simulink model "z_Ralenti_BO_End"  (R2024b)
settings: Solver=VariableStepAuto  StartTime=0.0  StopTime=10.0  RelTol=1e-3
undefined symbols (not defined in the file): AaNeTest, AAopti, Copti, gam, J, Kv, Mim0, N0, NeTest, NeTimeTest, nv_remp, P0, Pamb, PcolNeTest, PRcrit, Rair, SectionBpNeTest, table_rdt_AA, Tamb, Vcyl, vect_delta_AA
settings Model: Creator=a030141  LastModifiedBy=ramse
settings DebuggingCC: UnderspecifiedInitializationDetection=Classic  MergeDetectMultiDrivingBlocksExec=none
settings ModelReferenceCC: PropagateSignalLabelsOutOfModel=off

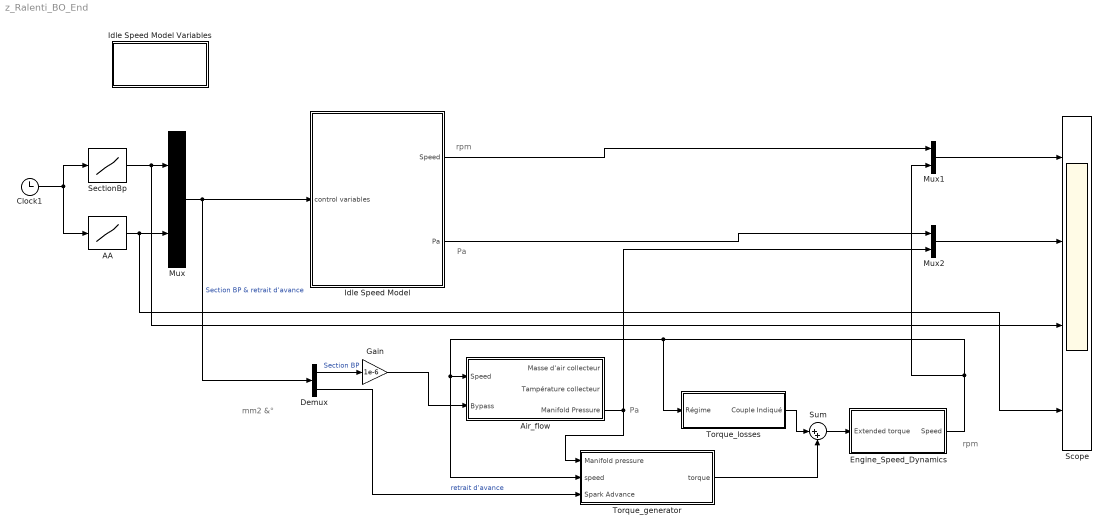
== system z_Ralenti_BO_End ==
  note: Pa
  note: rpm
  note: mm2 &°
  note: rpm
  note: Pa
  AA : Lookup  InputValues=NeTimeTest  Table=AaNeTest
  Air_flow : Subsystem
  Clock1 : Clock
  Demux : Demux  Outputs=2
  Engine_Speed_Dynamics : Subsystem
  Gain : Gain  Gain=1e-6
  Idle Speed Model : Subsystem
      mask Display: disp('ENGINE MODEL\nLF -> event stroke')
  Idle Speed Model Variables : Subsystem
      mask Display: disp('Load\nDisturbances')
  Mux : Mux  Inputs=2
      settings: DisplayOption=signals
  Mux1 : Mux  Inputs=2
  Mux2 : Mux  Inputs=2
  Scope : Scope  NumInputPorts=4
  SectionBp : Lookup  InputValues=NeTimeTest  Table=SectionBpNeTest
  Sum : Sum  Inputs=|++
  Torque_generator : Subsystem
  Torque_losses : Subsystem
  wires:
  Mux/1 -> Idle Speed Model/1(control variables), Demux/1  "Section BP & retrait d'avance"
  SectionBp/1 -> Mux/1, Scope/3
  AA/1 -> Mux/2, Scope/4
  Clock1/1 -> SectionBp/1, AA/1
  Idle Speed Model/1(Speed) -> Mux1/1
  Mux1/1 -> Scope/1
  Idle Speed Model/2(Pa) -> Mux2/1
  Mux2/1 -> Scope/2
  Demux/1 -> Gain/1  "Section BP"
  Demux/2 -> Torque_generator/3(Spark Advance)  "retrait d'avance"
  Air_flow/3(Manifold Pressure) -> Torque_generator/1(Manifold pressure), Mux2/2
  Engine_Speed_Dynamics/1(Speed) -> Mux1/2, Torque_losses/1(Régime), Torque_generator/2(speed), Air_flow/1(Speed)
  Gain/1 -> Air_flow/2(Bypass)
  Torque_losses/1(Couple Indiqué) -> Sum/1
  Torque_generator/1(torque) -> Sum/2
  Sum/1 -> Engine_Speed_Dynamics/1(Extended torque)

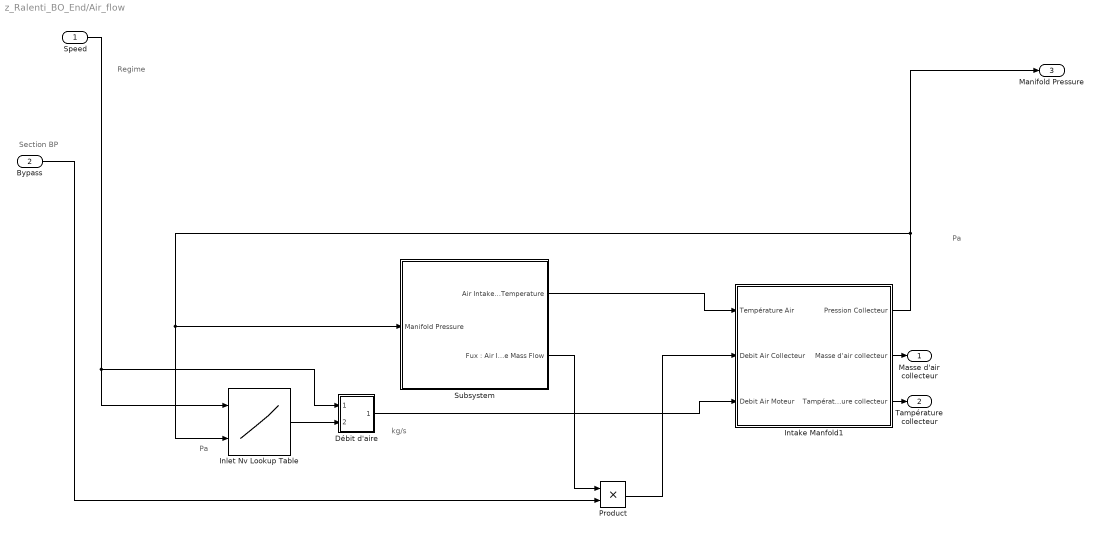
== system z_Ralenti_BO_End/Air_flow ==
  note: Section BP
  note: Regime
  note: Pa
  note: Pa
  note: kg/s
  Speed : Inport
  Bypass : Inport  Port=2
  Débit d'aire : Subsystem
  Inlet Nv Lookup Table : Lookup2D  RowIndex=Ne_remp  ColumnIndex=Pcol_remp  Table=nv_remp
  Intake Manfold1 : Subsystem
  Product : Product
  Subsystem : Subsystem
  Masse d'air collecteur : Outport
  Tampérature collecteur : Outport  Port=2
  Manifold Pressure : Outport  Port=3
  wires:
  Débit d'aire/1(Debit Air Moteur) -> Intake Manfold1/3(Debit Air Moteur)
  Speed/1 -> Débit d'aire/1(In1), Inlet Nv Lookup Table/1
  Intake Manfold1/2(Masse d'air collecteur) -> Masse d'air collecteur/1
  Subsystem/1(Air Intake Temperature) -> Intake Manfold1/1(Température Air)
  Subsystem/2("Fux : Air Intake Mass Flow") -> Product/1
  Inlet Nv Lookup Table/1 -> Débit d'aire/2(In2)
  Product/1 -> Intake Manfold1/2(Debit Air Collecteur)
  Intake Manfold1/1(Pression Collecteur) -> Manifold Pressure/1, Inlet Nv Lookup Table/2, Subsystem/1(Manifold Pressure)
  Bypass/1 -> Product/2
  Intake Manfold1/3(Tampérature collecteur) -> Tampérature collecteur/1

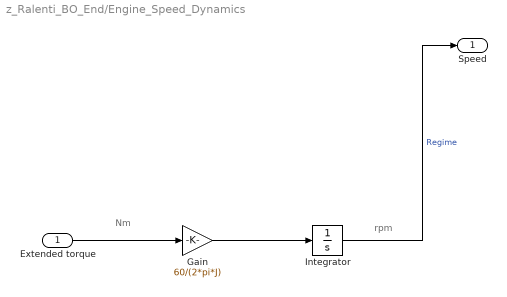
== system z_Ralenti_BO_End/Engine_Speed_Dynamics ==
  note: rpm
  note: Nm
  Extended torque : Inport
  Gain : Gain  Gain=60/(2*pi*J)
  Integrator : Integrator  InitialCondition=N0
  Speed : Outport
  wires:
  Gain/1 -> Integrator/1
  Extended torque/1 -> Gain/1
  Integrator/1 -> Speed/1  "Regime"

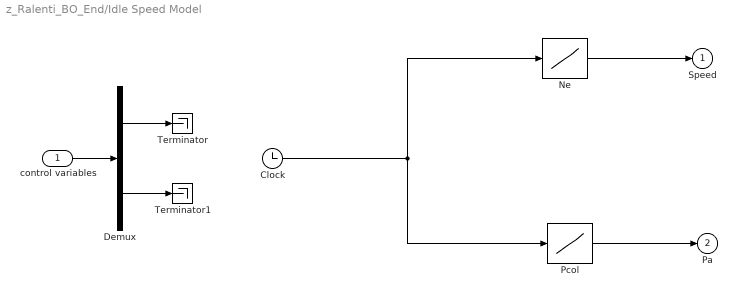
== system z_Ralenti_BO_End/Idle Speed Model ==
  control variables : Inport
  Clock : Clock
  Demux : Demux  Outputs=2
      settings: DisplayOption=none
  Ne : Lookup  InputValues=NeTimeTest  Table=NeTest
  Pcol : Lookup  InputValues=NeTimeTest  Table=PcolNeTest
  Terminator : Terminator
  Terminator1 : Terminator
  Speed : Outport
  Pa : Outport  Port=2
  wires:
  Demux/1 -> Terminator/1
  control variables/1 -> Demux/1
  Ne/1 -> Speed/1
  Pcol/1 -> Pa/1
  Clock/1 -> Ne/1, Pcol/1
  Demux/2 -> Terminator1/1

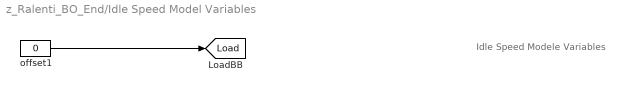
== system z_Ralenti_BO_End/Idle Speed Model Variables ==
  note: Idle Speed Modele Variables
  offset1 : Constant  Value=0
  tag scope: Load=global
  wires:
  offset1/1 -> [Load]

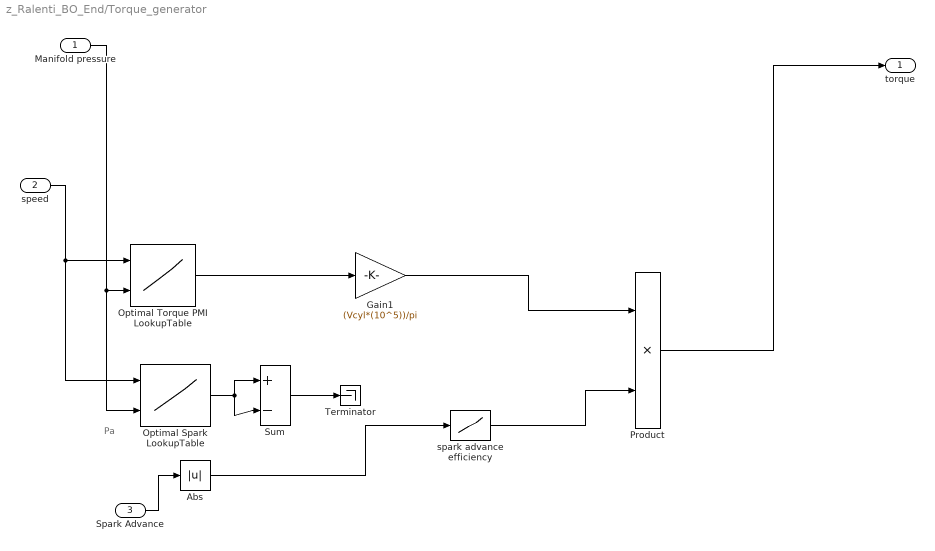
== system z_Ralenti_BO_End/Torque_generator ==
  note: Pa
  Manifold pressure : Inport
  speed : Inport  Port=2
  Spark Advance : Inport  Port=3
  Abs : Abs  SaturateOnIntegerOverflow=off
  Gain1 : Gain  Gain=(Vcyl*(10^5))/pi
  Optimal Spark LookupTable : Lookup2D  RowIndex=Ne_remp  ColumnIndex=Pcol_remp  Table=AAopti
  Optimal Torque PMI LookupTable : Lookup2D  RowIndex=Ne_remp  ColumnIndex=Pcol_remp  Table=Copti
  Product : Product
  Sum : Sum  Inputs=|+-
  Terminator : Terminator
  spark advance efficiency : Lookup  InputValues=vect_delta_AA  Table=table_rdt_AA
  torque : Outport
  wires:
  spark advance efficiency/1 -> Product/2
  speed/1 -> Optimal Spark LookupTable/1, Optimal Torque PMI LookupTable/1
  Gain1/1 -> Product/1
  Abs/1 -> spark advance efficiency/1
  Optimal Spark LookupTable/1 -> Sum/2, Sum/1
  Optimal Torque PMI LookupTable/1 -> Gain1/1
  Manifold pressure/1 -> Optimal Spark LookupTable/2, Optimal Torque PMI LookupTable/2
  Sum/1 -> Terminator/1
  Product/1 -> torque/1
  Spark Advance/1 -> Abs/1

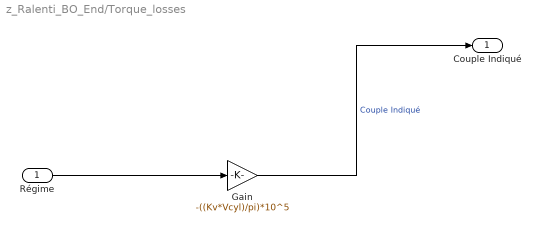
== system z_Ralenti_BO_End/Torque_losses ==
  Régime : Inport
  Gain : Gain  Gain=-((Kv*Vcyl)/pi)*10^5
  Couple Indiqué : Outport
  wires:
  Régime/1 -> Gain/1
  Gain/1 -> Couple Indiqué/1  "Couple Indiqué"

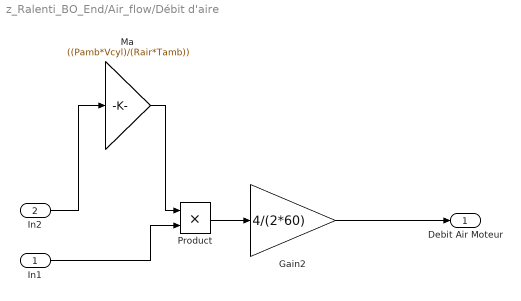
== system z_Ralenti_BO_End/Air_flow/Débit d'aire ==
  In1 : Inport
  In2 : Inport  Port=2
  Gain2 : Gain  Gain=4/(2*60)
  Ma : Gain  Gain=((Pamb*Vcyl)/(Rair*Tamb))
  Product : Product
  Debit Air Moteur : Outport
  wires:
  Ma/1 -> Product/1
  Gain2/1 -> Debit Air Moteur/1
  Product/1 -> Gain2/1
  In1/1 -> Product/2
  In2/1 -> Ma/1

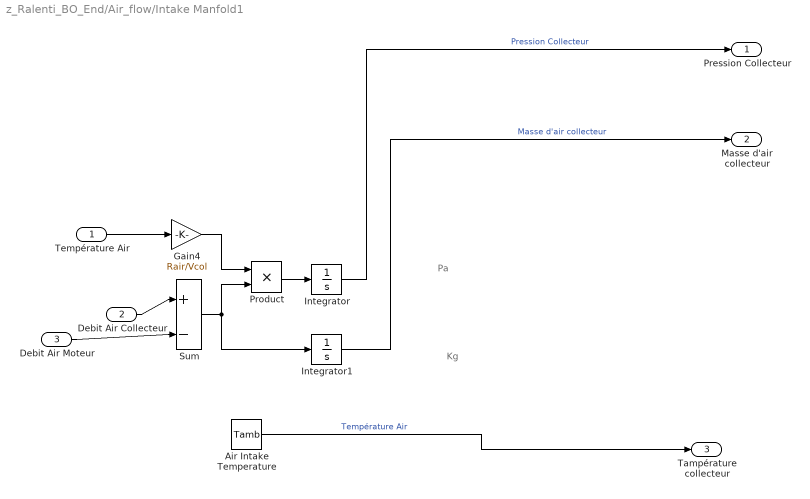
== system z_Ralenti_BO_End/Air_flow/Intake Manfold1 ==
  note: Pa
  note: Kg
  Température Air : Inport
  Debit Air Collecteur : Inport  Port=2
  Debit Air Moteur : Inport  Port=3
  Air Intake Temperature : Constant  Value=Tamb
  Gain4 : Gain  Gain=Rair/Vcol
  Integrator : Integrator  InitialCondition=P0
  Integrator1 : Integrator  InitialCondition=Mim0
  Product : Product
  Sum : Sum  Inputs=|+-
  Pression Collecteur : Outport
  Masse d'air collecteur : Outport  Port=2
  Tampérature collecteur : Outport  Port=3
  wires:
  Gain4/1 -> Product/1
  Sum/1 -> Integrator1/1, Product/2
  Product/1 -> Integrator/1
  Température Air/1 -> Gain4/1
  Integrator1/1 -> Masse d'air collecteur/1  "Masse d'air collecteur"
  Debit Air Moteur/1 -> Sum/2
  Integrator/1 -> Pression Collecteur/1  "Pression Collecteur"
  Debit Air Collecteur/1 -> Sum/1
  Air Intake Temperature/1 -> Tampérature collecteur/1  "Température Air"

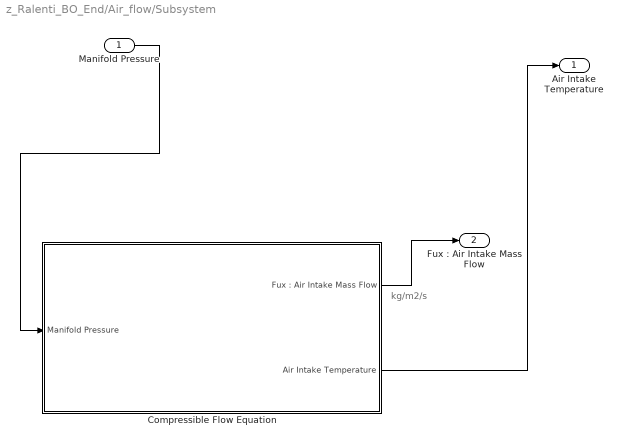
== system z_Ralenti_BO_End/Air_flow/Subsystem ==
  note: kg/m2/s
  Manifold Pressure : Inport
  Compressible Flow Equation : Subsystem
  Air Intake Temperature : Outport
  "Fux : Air Intake Mass Flow" : Outport  Port=2
  wires:
  Compressible Flow Equation/2(Air Intake Temperature) -> Air Intake Temperature/1
  Manifold Pressure/1 -> Compressible Flow Equation/1(Manifold Pressure)
  Compressible Flow Equation/1("Fux : Air Intake Mass Flow") -> "Fux : Air Intake Mass Flow"/1

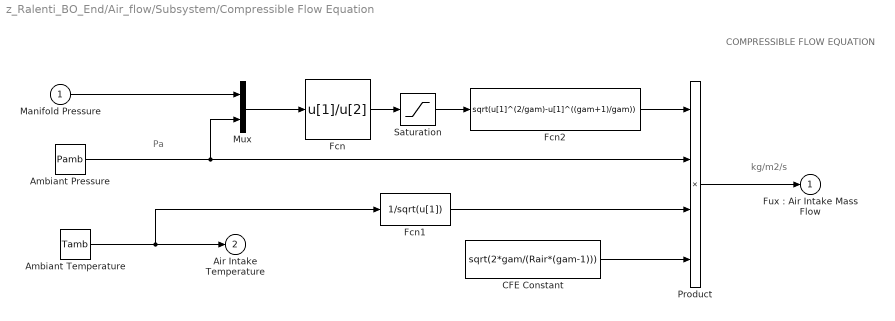
== system z_Ralenti_BO_End/Air_flow/Subsystem/Compressible Flow Equation ==
  note: COMPRESSIBLE FLOW EQUATION
  note: Pa
  note: kg/m2/s
  Manifold Pressure : Inport
  Ambiant Pressure : Constant  Value=Pamb
  Ambiant Temperature : Constant  Value=Tamb
  "CFE Constant " : Constant  Value=sqrt(2*gam/(Rair*(gam-1)))
  Fcn : Fcn  Expr=u[1]/u[2]
  Fcn1 : Fcn  Expr=1/sqrt(u[1])
  Fcn2 : Fcn  Expr=sqrt(u[1]^(2/gam)-u[1]^((gam+1)/gam))
  Mux : Mux  Inputs=2
  Product : Product  Inputs=4  InputSameDT=on  SaturateOnIntegerOverflow=on  OutDataTypeStr=Inherit: Same as first input
  Saturation : Saturate  UpperLimit=1  LowerLimit=PRcrit
  "Fux : Air Intake Mass Flow" : Outport
  Air Intake Temperature : Outport  Port=2
  wires:
  Ambiant Pressure/1 -> Product/2, Mux/2
  Product/1 -> "Fux : Air Intake Mass Flow"/1
  "CFE Constant "/1 -> Product/4
  Fcn2/1 -> Product/1
  Saturation/1 -> Fcn2/1
  Fcn1/1 -> Product/3
  Fcn/1 -> Saturation/1
  Mux/1 -> Fcn/1
  Manifold Pressure/1 -> Mux/1
  Ambiant Temperature/1 -> Fcn1/1, Air Intake Temperature/1
